simulink model "sudarshan_1 (2)"  (R2022b)
settings: Solver=ode4  StartTime=0.0  StopTime=1  FixedStep=0.0001  RelTol=1e-3
settings Model: Creator=year2  LastModifiedBy=year2

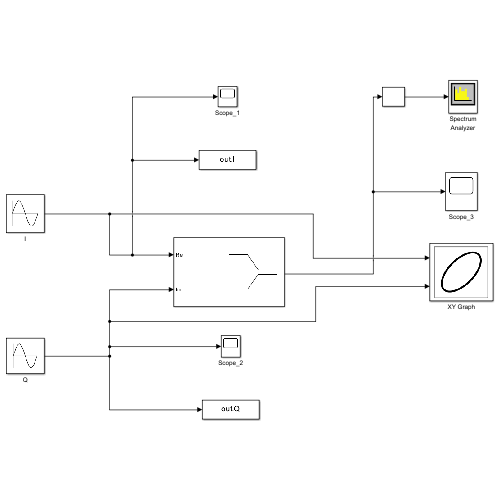
[thumbnail: Simulink's stored preview of the top-level diagram]
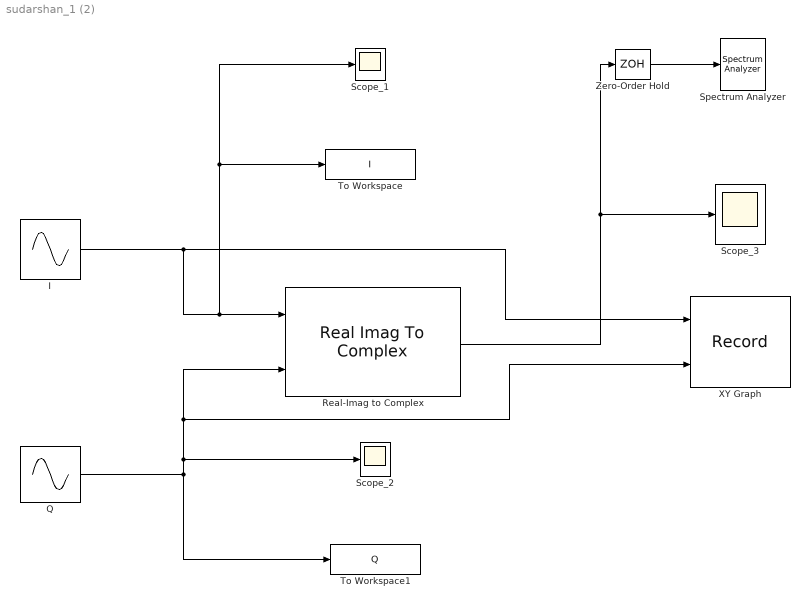
== system sudarshan_1 (2) ==
  I : Sin  Frequency=100  Phase=pi/2  SampleTime=0
  Q : Sin  Frequency=100  SampleTime=0
  Real-Imag to Complex : RealImagToComplex
  Scope_1 : Scope
  Scope_2 : Scope
  Scope_3 : Scope
  Spectrum Analyzer : SpectrumAnalyzer
  To Workspace : ToWorkspace  VariableName=I  SaveFormat=Timeseries  SampleTime=-1
  To Workspace1 : ToWorkspace  VariableName=Q  SaveFormat=Timeseries  SampleTime=-1
  XY Graph : Record  FileSettingsInternal="{\"entries\":[{\"content\":{\"excelSettings\":{\"content\":{},\"type\":\"Streamout.ExcelSettings\"}},\"type\":\"Streamout.FileSettingStorage\",\"uuid\":\"9869a838-1e5d-41e2-a3ef-ea152b2475d8\"}],\"packageUris\":[\"http://schema.mathworks.com/mf0/streamout_blocks/R2020a\"],\"version\":\"1.0\"}"  Layout=[1 1]  SignalsInternal="{\"entries\":[{\"content\":{\"signals\":[{\"content\":{\"blockPath\":[\"sudarshan_1/XY Graph\"],\"channel\":[],\"dimensions\":[1],\"domain\":\"sudarshan_1/XY Graph\",\"lineColor\":\"#a2142f\",\"plots\":[1],\"port\":1,\"sid\":[\"\"],\"signalID\":863,\"signalName\":\"I\"},\"type\":\"RecordBlkView.Signal\",\"uuid\":\"b3831935-c9d8-4619-b58c-8d1a0a993c52\"},{\"content\":{\"blockPath\":[\"sudarshan_1/XY Graph\"],\"channel\":[],\"dimensions\":[1],\"domain\":\"sudarshan_1/XY Graph\",\"lineColor\":\"#139fff\",\"plots\":[1],\"port\":2,\"sid\":[\"\"],\"signalID\":867,\"signalName\":\"Q\"},\"type\":\"RecordBlkView.Signal\",\"uuid\":\"725f82f0-ebd8-429a-aded-21ad64571e3d\"}]},\"type\":\"RecordBlkView.InputSignals\",\"uuid\":\"01d4348e-3a75-4d5c-bb24-ad9471c30897\"}],\"packageUris\":[\"http://schema.mathworks.com/mf0/streamout_blocks/R2020a\"],\"version\":\"1.0\"}"  VisualizationBindings="{\"xyplotplugin\":{\"info\":[{\"series\":[{\"bindingParametersList\":[{\"parameter\":\"X-Axis\",\"signalID\":863,\"signalName\":\"I\"},{\"parameter\":\"Y-Axis\",\"signalID\":867,\"signalName\":\"Q\"}],\"seriesID\":43396}],\"subplotID\":1}]}}"  CompatibilityTag=XY  st=-1
  Zero-Order Hold : ZeroOrderHold  SampleTime=-1
  wires:
  Q/1 -> To Workspace1/1, XY Graph/2, Real-Imag to Complex/2, Scope_2/1
  I/1 -> XY Graph/1, To Workspace/1, Scope_1/1, Real-Imag to Complex/1
  Real-Imag to Complex/1 -> Scope_3/1, Zero-Order Hold/1
  Zero-Order Hold/1 -> Spectrum Analyzer/1
